simulink model "test_myverify"  (R2019a)
settings: Solver=VariableStepAuto  StartTime=0.0  StopTime=10.0  RelTol=1e-3
values from neighbouring files (symbols this model uses):
  delta = 1    [tset_1.m]
  den = [1 1]    [tset_1.m]
  num = [1]    [tset_1.m]
libraries: slident x1
settings Model: Creator=lzr96  LastModifiedBy=lzr96

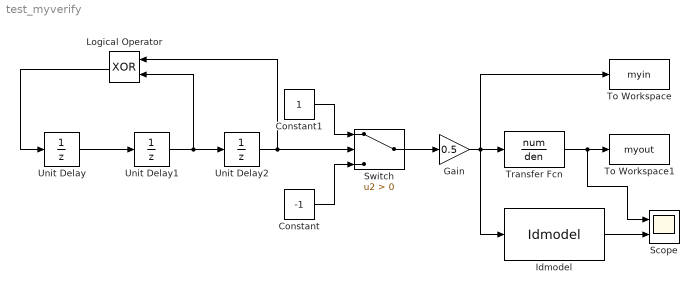
== system test_myverify ==
  Constant : Constant  Value=-1
  Constant1 : Constant
  Gain : Gain  Gain=0.5
  Idmodel : slident/Models/Idmodel  sys=Model  IC=0  noi=on  seed=[]
      settings: SourceProductName=System Identification Toolbox  SourceProductBaseCode=ID
  Logical Operator : Logic  Operator=XOR  AllPortsSameDT=off  OutDataTypeStr=boolean
  Scope : Scope  NumInputPorts=2
  Switch : Switch  Criteria=u2 > Threshold
  To Workspace : ToWorkspace  VariableName=myin  SampleTime=delta
  To Workspace1 : ToWorkspace  VariableName=myout  SampleTime=delta
  Transfer Fcn : TransferFcn  Numerator=num  Denominator=den
  Unit Delay : UnitDelay  SampleTime=delta  HasFrameUpgradeWarning=on
  Unit Delay1 : UnitDelay  InitialCondition=1  SampleTime=delta  HasFrameUpgradeWarning=on
  Unit Delay2 : UnitDelay  SampleTime=delta  HasFrameUpgradeWarning=on
  wires:
  Idmodel/1 -> Scope/2
  Constant1/1 -> Switch/1
  Transfer Fcn/1 -> Scope/1, To Workspace1/1
  Gain/1 -> Idmodel/1, To Workspace/1, Transfer Fcn/1
  Constant/1 -> Switch/3
  Unit Delay2/1 -> Logical Operator/1, Switch/2
  Unit Delay1/1 -> Logical Operator/2, Unit Delay2/1
  Unit Delay/1 -> Unit Delay1/1
  Switch/1 -> Gain/1
  Logical Operator/1 -> Unit Delay/1
